simulink model "f2"  (R2014a)
settings: Solver=ode45  StartTime=0.0  StopTime=10  RelTol=1e-3
settings Model: Creator=root  LastModifiedBy=root

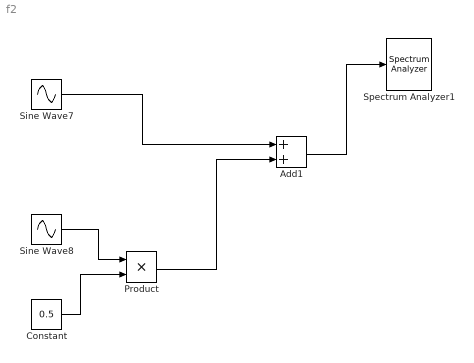
== system f2 ==
  Add1 : Sum
  Constant : Constant  Value=0.5
  Product : Product
  Sine Wave7 : Sin  Frequency=200*pi  Phase=pi/2  SampleTime=0.001
  Sine Wave8 : Sin  Frequency=20*pi  Phase=pi/2  SampleTime=0.001
  Spectrum Analyzer1 : SpectrumAnalyzer
  wires:
  Sine Wave8/1 -> Product/1
  Constant/1 -> Product/2
  Product/1 -> Add1/2
  Sine Wave7/1 -> Add1/1
  Add1/1 -> Spectrum Analyzer1/1
